simulink model "SolarSimulation"  (R2018b)
settings: Solver=VariableStepAuto  StartTime=0.0  StopTime=10.0  RelTol=1e-3
libraries: elec_lib x486, nesl_utility x22, fl_lib x7, simulink x2
(part 2 of 2)

== system SolarSimulation/Whole Panel/27 cell strip 6 ==
  Solar Irradiance : Inport
  Simulink-PS Converter : nesl_utility/Simulink-PS Converter  PhysicalDomain=network_engine_domain  SubClassName=ps_input  LeftPortType=input  RightPortType=output  PseudoPeriodic=off  Frequencies=[]  NoiseDistribution=none  NoiseParameters=[]  Unit=1  AffineConversion=off  FilteringAndDerivatives=provide  SimscapeFilterOrder=1  InputFilterTimeConstant=0.001  UdotUserProvided=0
  Solar Cell{,1..26} (27 alike) : elec_lib/Sources/Solar Cell  prm=1  Isc=1.55 A  Voc=.668 V  Is=1.39E-11 A  Is2=4.1866E-7 A  Iph=1.55 A  Ir0=1000 W/m^2  ec=1.022  N2=1.022  Rs="0.017   Ohm"  Rp=263 Ohm  N_series=1  TIPH1="0.0003551  1/K"  EG=1.166 eV  TXIS1=3  TXIS2=3  TRS1=0  TRP1=0  Tmeas=25 degC  TFIXED=25 degC  thermal_mass=100 J/K  initial_temperature=25 degC
      settings: SourceProductName=Simscape Electronics  SourceProductBaseCode=SN
  + : PMIOPort  Side=Left
  - : PMIOPort  Port=2  Side=Left
  wires:
  Solar Irradiance/1 -> Simulink-PS Converter/1
  connections:
  Solar Cell5/LConn2 -- Solar Cell4/RConn1
  Solar Cell26/LConn1 -- Solar Cell24/LConn1 -- Solar Cell23/LConn1 -- Solar Cell22/LConn1 -- Solar Cell21/LConn1 -- Solar Cell20/LConn1 -- Solar Cell19/LConn1 -- Solar Cell18/LConn1 -- Solar Cell9/LConn1 -- Solar Cell1/LConn1 -- Solar Cell2/LConn1 -- Solar Cell3/LConn1 -- Solar Cell4/LConn1 -- Solar Cell5/LConn1 -- Solar Cell6/LConn1 -- Solar Cell8/LConn1 -- Solar Cell7/LConn1 -- Simulink-PS Converter/RConn1 -- Solar Cell/LConn1 -- Solar Cell10/LConn1 -- Solar Cell11/LConn1 -- Solar Cell12/LConn1 -- Solar Cell13/LConn1 -- Solar Cell14/LConn1 -- Solar Cell15/LConn1 -- Solar Cell17/LConn1 -- Solar Cell16/LConn1 -- Solar Cell25/LConn1
  Solar Cell1/LConn2 -- Solar Cell/RConn1
  Solar Cell2/LConn2 -- Solar Cell1/RConn1
  Solar Cell6/LConn2 -- Solar Cell5/RConn1
  Solar Cell8/LConn2 -- Solar Cell7/RConn1
  Solar Cell4/LConn2 -- Solar Cell3/RConn1
  Solar Cell7/LConn2 -- Solar Cell6/RConn1
  +/RConn1 -- Solar Cell/LConn2
  Solar Cell3/LConn2 -- Solar Cell2/RConn1
  Solar Cell16/LConn2 -- Solar Cell15/RConn1
  Solar Cell12/RConn1 -- Solar Cell13/LConn2
  Solar Cell15/LConn2 -- Solar Cell14/RConn1
  Solar Cell17/LConn2 -- Solar Cell16/RConn1
  Solar Cell12/LConn2 -- Solar Cell11/RConn1
  Solar Cell14/LConn2 -- Solar Cell13/RConn1
  Solar Cell9/RConn1 -- Solar Cell10/LConn2
  Solar Cell10/RConn1 -- Solar Cell11/LConn2
  Solar Cell22/RConn1 -- Solar Cell23/LConn2
  Solar Cell21/LConn2 -- Solar Cell20/RConn1
  Solar Cell18/RConn1 -- Solar Cell19/LConn2
  Solar Cell24/LConn2 -- Solar Cell23/RConn1
  Solar Cell19/RConn1 -- Solar Cell20/LConn2
  Solar Cell25/RConn1 -- Solar Cell26/LConn2
  Solar Cell25/LConn2 -- Solar Cell24/RConn1
  Solar Cell21/RConn1 -- Solar Cell22/LConn2
  Solar Cell9/LConn2 -- Solar Cell8/RConn1
  Solar Cell18/LConn2 -- Solar Cell17/RConn1
  Solar Cell26/RConn1 -- -/RConn1

== system SolarSimulation/Whole Panel/27 cell strip 7 ==
  Solar Irradiance : Inport
  Simulink-PS Converter : nesl_utility/Simulink-PS Converter  PhysicalDomain=network_engine_domain  SubClassName=ps_input  LeftPortType=input  RightPortType=output  PseudoPeriodic=off  Frequencies=[]  NoiseDistribution=none  NoiseParameters=[]  Unit=1  AffineConversion=off  FilteringAndDerivatives=provide  SimscapeFilterOrder=1  InputFilterTimeConstant=0.001  UdotUserProvided=0
  Solar Cell{,1..26} (27 alike) : elec_lib/Sources/Solar Cell  prm=1  Isc=1.55 A  Voc=.668 V  Is=1.39E-11 A  Is2=4.1866E-7 A  Iph=1.55 A  Ir0=1000 W/m^2  ec=1.022  N2=1.022  Rs="0.017   Ohm"  Rp=263 Ohm  N_series=1  TIPH1="0.0003551  1/K"  EG=1.166 eV  TXIS1=3  TXIS2=3  TRS1=0  TRP1=0  Tmeas=25 degC  TFIXED=25 degC  thermal_mass=100 J/K  initial_temperature=25 degC
      settings: SourceProductName=Simscape Electronics  SourceProductBaseCode=SN
  + : PMIOPort  Side=Left
  - : PMIOPort  Port=2  Side=Left
  wires:
  Solar Irradiance/1 -> Simulink-PS Converter/1
  connections:
  Solar Cell5/LConn2 -- Solar Cell4/RConn1
  Solar Cell26/LConn1 -- Solar Cell24/LConn1 -- Solar Cell23/LConn1 -- Solar Cell22/LConn1 -- Solar Cell21/LConn1 -- Solar Cell20/LConn1 -- Solar Cell19/LConn1 -- Solar Cell18/LConn1 -- Solar Cell9/LConn1 -- Solar Cell1/LConn1 -- Solar Cell2/LConn1 -- Solar Cell3/LConn1 -- Solar Cell4/LConn1 -- Solar Cell5/LConn1 -- Solar Cell6/LConn1 -- Solar Cell8/LConn1 -- Solar Cell7/LConn1 -- Simulink-PS Converter/RConn1 -- Solar Cell/LConn1 -- Solar Cell10/LConn1 -- Solar Cell11/LConn1 -- Solar Cell12/LConn1 -- Solar Cell13/LConn1 -- Solar Cell14/LConn1 -- Solar Cell15/LConn1 -- Solar Cell17/LConn1 -- Solar Cell16/LConn1 -- Solar Cell25/LConn1
  Solar Cell1/LConn2 -- Solar Cell/RConn1
  Solar Cell2/LConn2 -- Solar Cell1/RConn1
  Solar Cell6/LConn2 -- Solar Cell5/RConn1
  Solar Cell8/LConn2 -- Solar Cell7/RConn1
  Solar Cell4/LConn2 -- Solar Cell3/RConn1
  Solar Cell7/LConn2 -- Solar Cell6/RConn1
  +/RConn1 -- Solar Cell/LConn2
  Solar Cell3/LConn2 -- Solar Cell2/RConn1
  Solar Cell16/LConn2 -- Solar Cell15/RConn1
  Solar Cell12/RConn1 -- Solar Cell13/LConn2
  Solar Cell15/LConn2 -- Solar Cell14/RConn1
  Solar Cell17/LConn2 -- Solar Cell16/RConn1
  Solar Cell12/LConn2 -- Solar Cell11/RConn1
  Solar Cell14/LConn2 -- Solar Cell13/RConn1
  Solar Cell9/RConn1 -- Solar Cell10/LConn2
  Solar Cell10/RConn1 -- Solar Cell11/LConn2
  Solar Cell22/RConn1 -- Solar Cell23/LConn2
  Solar Cell21/LConn2 -- Solar Cell20/RConn1
  Solar Cell18/RConn1 -- Solar Cell19/LConn2
  Solar Cell24/LConn2 -- Solar Cell23/RConn1
  Solar Cell19/RConn1 -- Solar Cell20/LConn2
  Solar Cell25/RConn1 -- Solar Cell26/LConn2
  Solar Cell25/LConn2 -- Solar Cell24/RConn1
  Solar Cell21/RConn1 -- Solar Cell22/LConn2
  Solar Cell9/LConn2 -- Solar Cell8/RConn1
  Solar Cell18/LConn2 -- Solar Cell17/RConn1
  Solar Cell26/RConn1 -- -/RConn1

== system SolarSimulation/Whole Panel/27 cell strip 8 ==
  Solar Irradiance : Inport
  Simulink-PS Converter : nesl_utility/Simulink-PS Converter  PhysicalDomain=network_engine_domain  SubClassName=ps_input  LeftPortType=input  RightPortType=output  PseudoPeriodic=off  Frequencies=[]  NoiseDistribution=none  NoiseParameters=[]  Unit=1  AffineConversion=off  FilteringAndDerivatives=provide  SimscapeFilterOrder=1  InputFilterTimeConstant=0.001  UdotUserProvided=0
  Solar Cell{,1..26} (27 alike) : elec_lib/Sources/Solar Cell  prm=1  Isc=1.55 A  Voc=.668 V  Is=1.39E-11 A  Is2=4.1866E-7 A  Iph=1.55 A  Ir0=1000 W/m^2  ec=1.022  N2=1.022  Rs="0.017   Ohm"  Rp=263 Ohm  N_series=1  TIPH1="0.0003551  1/K"  EG=1.166 eV  TXIS1=3  TXIS2=3  TRS1=0  TRP1=0  Tmeas=25 degC  TFIXED=25 degC  thermal_mass=100 J/K  initial_temperature=25 degC
      settings: SourceProductName=Simscape Electronics  SourceProductBaseCode=SN
  + : PMIOPort  Side=Left
  - : PMIOPort  Port=2  Side=Left
  wires:
  Solar Irradiance/1 -> Simulink-PS Converter/1
  connections:
  Solar Cell5/LConn2 -- Solar Cell4/RConn1
  Solar Cell26/LConn1 -- Solar Cell24/LConn1 -- Solar Cell23/LConn1 -- Solar Cell22/LConn1 -- Solar Cell21/LConn1 -- Solar Cell20/LConn1 -- Solar Cell19/LConn1 -- Solar Cell18/LConn1 -- Solar Cell9/LConn1 -- Solar Cell1/LConn1 -- Solar Cell2/LConn1 -- Solar Cell3/LConn1 -- Solar Cell4/LConn1 -- Solar Cell5/LConn1 -- Solar Cell6/LConn1 -- Solar Cell8/LConn1 -- Solar Cell7/LConn1 -- Simulink-PS Converter/RConn1 -- Solar Cell/LConn1 -- Solar Cell10/LConn1 -- Solar Cell11/LConn1 -- Solar Cell12/LConn1 -- Solar Cell13/LConn1 -- Solar Cell14/LConn1 -- Solar Cell15/LConn1 -- Solar Cell17/LConn1 -- Solar Cell16/LConn1 -- Solar Cell25/LConn1
  Solar Cell1/LConn2 -- Solar Cell/RConn1
  Solar Cell2/LConn2 -- Solar Cell1/RConn1
  Solar Cell6/LConn2 -- Solar Cell5/RConn1
  Solar Cell8/LConn2 -- Solar Cell7/RConn1
  Solar Cell4/LConn2 -- Solar Cell3/RConn1
  Solar Cell7/LConn2 -- Solar Cell6/RConn1
  +/RConn1 -- Solar Cell/LConn2
  Solar Cell3/LConn2 -- Solar Cell2/RConn1
  Solar Cell16/LConn2 -- Solar Cell15/RConn1
  Solar Cell12/RConn1 -- Solar Cell13/LConn2
  Solar Cell15/LConn2 -- Solar Cell14/RConn1
  Solar Cell17/LConn2 -- Solar Cell16/RConn1
  Solar Cell12/LConn2 -- Solar Cell11/RConn1
  Solar Cell14/LConn2 -- Solar Cell13/RConn1
  Solar Cell9/RConn1 -- Solar Cell10/LConn2
  Solar Cell10/RConn1 -- Solar Cell11/LConn2
  Solar Cell22/RConn1 -- Solar Cell23/LConn2
  Solar Cell21/LConn2 -- Solar Cell20/RConn1
  Solar Cell18/RConn1 -- Solar Cell19/LConn2
  Solar Cell24/LConn2 -- Solar Cell23/RConn1
  Solar Cell19/RConn1 -- Solar Cell20/LConn2
  Solar Cell25/RConn1 -- Solar Cell26/LConn2
  Solar Cell25/LConn2 -- Solar Cell24/RConn1
  Solar Cell21/RConn1 -- Solar Cell22/LConn2
  Solar Cell9/LConn2 -- Solar Cell8/RConn1
  Solar Cell18/LConn2 -- Solar Cell17/RConn1
  Solar Cell26/RConn1 -- -/RConn1

== system SolarSimulation/Whole Panel/27 cell strip 9 ==
  Solar Irradiance : Inport
  Simulink-PS Converter : nesl_utility/Simulink-PS Converter  PhysicalDomain=network_engine_domain  SubClassName=ps_input  LeftPortType=input  RightPortType=output  PseudoPeriodic=off  Frequencies=[]  NoiseDistribution=none  NoiseParameters=[]  Unit=1  AffineConversion=off  FilteringAndDerivatives=provide  SimscapeFilterOrder=1  InputFilterTimeConstant=0.001  UdotUserProvided=0
  Solar Cell{,1..26} (27 alike) : elec_lib/Sources/Solar Cell  prm=1  Isc=1.55 A  Voc=.668 V  Is=1.39E-11 A  Is2=4.1866E-7 A  Iph=1.55 A  Ir0=1000 W/m^2  ec=1.022  N2=1.022  Rs="0.017   Ohm"  Rp=263 Ohm  N_series=1  TIPH1="0.0003551  1/K"  EG=1.166 eV  TXIS1=3  TXIS2=3  TRS1=0  TRP1=0  Tmeas=25 degC  TFIXED=25 degC  thermal_mass=100 J/K  initial_temperature=25 degC
      settings: SourceProductName=Simscape Electronics  SourceProductBaseCode=SN
  + : PMIOPort  Side=Left
  - : PMIOPort  Port=2  Side=Left
  wires:
  Solar Irradiance/1 -> Simulink-PS Converter/1
  connections:
  Solar Cell5/LConn2 -- Solar Cell4/RConn1
  Solar Cell26/LConn1 -- Solar Cell24/LConn1 -- Solar Cell23/LConn1 -- Solar Cell22/LConn1 -- Solar Cell21/LConn1 -- Solar Cell20/LConn1 -- Solar Cell19/LConn1 -- Solar Cell18/LConn1 -- Solar Cell9/LConn1 -- Solar Cell1/LConn1 -- Solar Cell2/LConn1 -- Solar Cell3/LConn1 -- Solar Cell4/LConn1 -- Solar Cell5/LConn1 -- Solar Cell6/LConn1 -- Solar Cell8/LConn1 -- Solar Cell7/LConn1 -- Simulink-PS Converter/RConn1 -- Solar Cell/LConn1 -- Solar Cell10/LConn1 -- Solar Cell11/LConn1 -- Solar Cell12/LConn1 -- Solar Cell13/LConn1 -- Solar Cell14/LConn1 -- Solar Cell15/LConn1 -- Solar Cell17/LConn1 -- Solar Cell16/LConn1 -- Solar Cell25/LConn1
  Solar Cell1/LConn2 -- Solar Cell/RConn1
  Solar Cell2/LConn2 -- Solar Cell1/RConn1
  Solar Cell6/LConn2 -- Solar Cell5/RConn1
  Solar Cell8/LConn2 -- Solar Cell7/RConn1
  Solar Cell4/LConn2 -- Solar Cell3/RConn1
  Solar Cell7/LConn2 -- Solar Cell6/RConn1
  +/RConn1 -- Solar Cell/LConn2
  Solar Cell3/LConn2 -- Solar Cell2/RConn1
  Solar Cell16/LConn2 -- Solar Cell15/RConn1
  Solar Cell12/RConn1 -- Solar Cell13/LConn2
  Solar Cell15/LConn2 -- Solar Cell14/RConn1
  Solar Cell17/LConn2 -- Solar Cell16/RConn1
  Solar Cell12/LConn2 -- Solar Cell11/RConn1
  Solar Cell14/LConn2 -- Solar Cell13/RConn1
  Solar Cell9/RConn1 -- Solar Cell10/LConn2
  Solar Cell10/RConn1 -- Solar Cell11/LConn2
  Solar Cell22/RConn1 -- Solar Cell23/LConn2
  Solar Cell21/LConn2 -- Solar Cell20/RConn1
  Solar Cell18/RConn1 -- Solar Cell19/LConn2
  Solar Cell24/LConn2 -- Solar Cell23/RConn1
  Solar Cell19/RConn1 -- Solar Cell20/LConn2
  Solar Cell25/RConn1 -- Solar Cell26/LConn2
  Solar Cell25/LConn2 -- Solar Cell24/RConn1
  Solar Cell21/RConn1 -- Solar Cell22/LConn2
  Solar Cell9/LConn2 -- Solar Cell8/RConn1
  Solar Cell18/LConn2 -- Solar Cell17/RConn1
  Solar Cell26/RConn1 -- -/RConn1
